simulink model "d_simulink"  (R2013a)
settings: Solver=VariableStepDiscrete  StartTime=0.0  StopTime=70  RelTol=1e-3
values from neighbouring files (symbols this model uses):
  a1 = a1_k    (= -1.686)    [d_generell.m]    (also in d_iterativ.m)
  a2 = a2_k    (= 0.7097)    [d_generell.m]    (also in d_iterativ.m)
  b3 = b3_k    (= 1.526e-06)    [d_generell.m]    (also in d_iterativ.m)
  b4 = b4_k    (= 1.361e-06)    [d_generell.m]    (also in d_iterativ.m)
  c1 = c1_k    [d_generell.m]    (also in d_iterativ.m = 1343/500 - 3*q)
  c2 = c2_k    [d_generell.m]    (also in d_iterativ.m = 3*q^2 - (4029*q)/500 + 301181/62500)
  c3 = c3_k    [d_generell.m]    (also in d_iterativ.m = -(1327466112874474796439510129852430213846220285015000*q^3)/)
  d0 = d0_k    [d_generell.m]    (also in d_iterativ.m = -(6110003985060045229383251247700656165922412773939236306944)
  d1 = d1_k    [d_generell.m]    (also in d_iterativ.m = (3112805664800708920027824490335592561049122132143974121472*)
  d2 = d2_k    [d_generell.m]    (also in d_iterativ.m = -(692213593171943264470864977050316873216081921657656049664*)
  Kr = double(subs(Kr, [b3 b4 q], [b3_k b4_k q_k]))    [d_generell.m]    (also in d_iterativ.m = -(2361183241434822606848*q^3)/6816736018022333 + (7083549724)
  Ku = 1/(Q*c*r)    (= 0.00011961722488)    [d_generell.m]
settings Model: Creator=Tobias  LastModifiedBy=Tobias

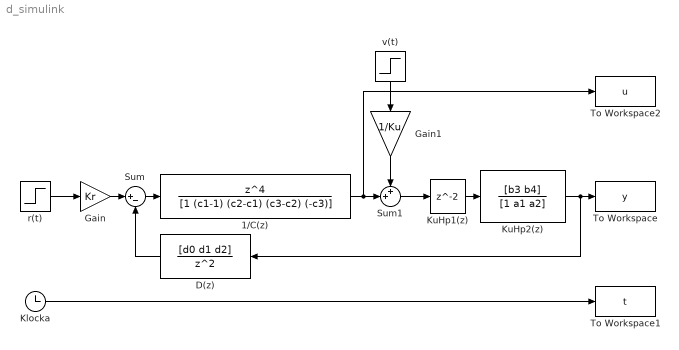
== system d_simulink ==
  1/C(z) : DiscreteTransferFcn  Numerator=[1 0 0 0 0]  Denominator=[1 (c1-1) (c2-c1) (c3-c2) (-c3)]
  D(z) : DiscreteTransferFcn  Numerator=[d0 d1 d2]  Denominator=[1 0 0]
  Gain : Gain  Gain=Kr
  Gain1 : Gain  Gain=1/Ku
  Klocka : Clock
  KuHp1(z) : Delay
  KuHp2(z) : DiscreteTransferFcn  Numerator=[b3 b4]  Denominator=[1 a1 a2]
  Sum : Sum  Inputs=|+-
  Sum1 : Sum  Inputs=++|
  To Workspace : ToWorkspace  VariableName=y  SampleTime=-1
  To Workspace1 : ToWorkspace  VariableName=t  SampleTime=-1
  To Workspace2 : ToWorkspace  VariableName=u  SampleTime=-1
  r(t) : Step  After=0  SampleTime=1
  v(t) : Step  SampleTime=1
  wires:
  KuHp1(z)/1 -> KuHp2(z)/1
  D(z)/1 -> Sum/2
  Gain/1 -> Sum/1
  Sum/1 -> 1/C(z)/1
  Sum1/1 -> KuHp1(z)/1
  Gain1/1 -> Sum1/1
  1/C(z)/1 -> To Workspace2/1, Sum1/2
  v(t)/1 -> Gain1/1
  r(t)/1 -> Gain/1
  KuHp2(z)/1 -> To Workspace/1, D(z)/1
  Klocka/1 -> To Workspace1/1
